simulink model "a_adaptivesInveresFilter"  (R2024b)
settings: Solver=ode45  StartTime=0.0  StopTime=100000.0  RelTol=1e-3  EnableMultiTasking=on
undefined symbols (not defined in the file): Amplitudengang, dspblkCoreblockFVToolHelper, gcbh, Koeffizienten, LMS, RLS
libraries: simulink x3, dspadpt3 x2, dspspect3 x2
settings Model: Creator=Wirnitzer  LastModifiedBy=49179
settings SolverCC: AlgebraicLoopSolver=TrustRegion
settings DataIOCC: LimitDataPoints=on  SaveFormat=Array  SignalLoggingSaveFormat=ModelDataLogs  ReturnWorkspaceOutputs=off
settings OptimizationCC: BooleanDataType=off  InitFltsAndDblsToZero=on  LifeSpan=inf
settings DebuggingCC: SaveWithParameterizedLinksMsg=none  UnderspecifiedInitializationDetection=Classic  MergeDetectMultiDrivingBlocksExec=none  SignalResolutionControl=TryResolveAllWithWarning  MultiTaskDSMMsg=warning  MultiTaskCondExecSysMsg=none  FcnCallInpInsideContextMsg=warning  UnconnectedInputMsg=warning  UnconnectedOutputMsg=warning  UnconnectedLineMsg=warning  SFUnexpectedBacktrackingDiag=warning  SFNoUnconditionalDefaultTransitionDiag=warning  SFExecutionAtInitializationDiag=none  ArithmeticOperatorsInVariantConditions=warning
settings HardwareCC: ProdBitPerPointer=32  ProdBitPerSizeT=32  ProdBitPerPtrDiffT=32  ProdLargestAtomicFloat=None  ProdIntDivRoundTo=Undefined  ProdEndianess=Unspecified  ProdWordSize=32  ProdHWDeviceType=32-bit Generic  TargetUnknown=on
settings ModelReferenceCC: EnableRefExpFcnMdlSchedulingChecks=on  PropagateSignalLabelsOutOfModel=off
settings SFSimCC: CustomCodeUndefinedFunction=UseInterfaceOnly
settings RTWCC: GPUComputeCapability=3.5
settings CodeAppCC: StateflowObjectComments=on
settings GRTTargetCC: TargetFcnLib=ansi_tfl_tmw.mat  TargetLangStandard=C89/C90 (ANSI)  ModelReferenceCompliant=off  CombineOutputUpdateFcns=off  MatFileLogging=off  GRTInterface=on
settings ConfigComp: CovMetricSettings=dw  CovSaveCumulativeToWorkspaceVar=on  CovSaveSingleToWorkspaceVar=on

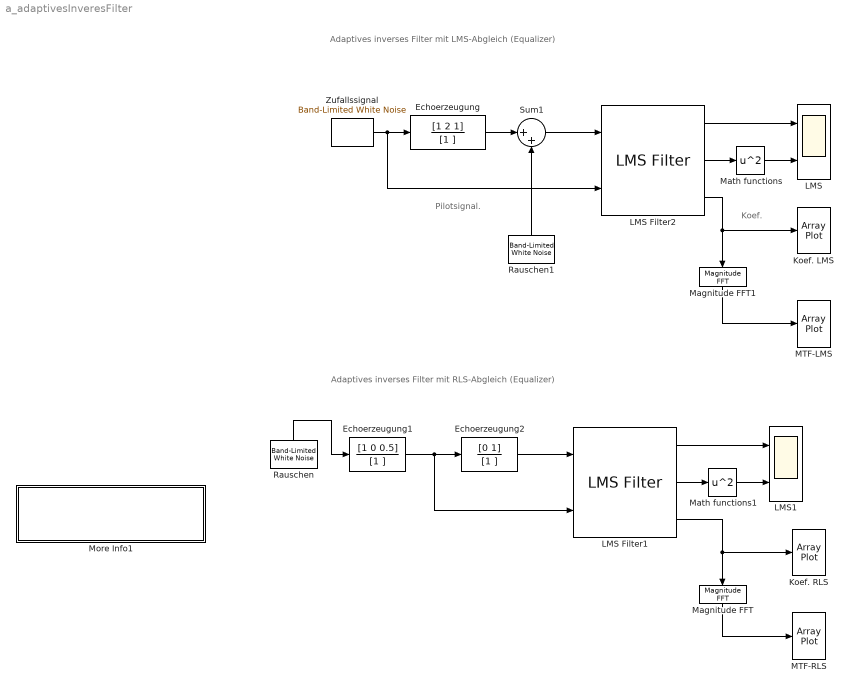
== system a_adaptivesInveresFilter ==
  note: Pilotsignal.
  note: Adaptives inverses  Filter mit RLS-Abgleich
      |  (Equalizer)
  note: Koef.
  note: Adaptives inverses  Filter mit LMS-Abgleich
      | (Equalizer)
  Echoerzeugung : DiscreteFilter  LoadFcn=dspblkCoreblockFVToolHelper(gcbh,'load');  Numerator=[1 2 1]  Denominator=[1 ]  SampleTime=1
      settings: CopyFcn=dspblkCoreblockFVToolHelper(gcbh,'copy');  DeleteFcn=dspblkCoreblockFVToolHelper(gcbh,'close');  ModelCloseFcn=dspblkCoreblockFVToolHelper(gcbh,'close');  PreSaveFcn=dspblkCoreblockFVToolHelper(gcbh,'presave');  PostSaveFcn=dspblkCoreblockFVToolHelper(gcbh,'postsave');  CloseFcn=dspblkCoreblockFVToolHelper(gcbh,'close');
  Echoerzeugung1 : DiscreteFilter  LoadFcn=dspblkCoreblockFVToolHelper(gcbh,'load');  Numerator=[1 0 0.5]  Denominator=[1 ]  SampleTime=1
      settings: CopyFcn=dspblkCoreblockFVToolHelper(gcbh,'copy');  DeleteFcn=dspblkCoreblockFVToolHelper(gcbh,'close');  ModelCloseFcn=dspblkCoreblockFVToolHelper(gcbh,'close');  PreSaveFcn=dspblkCoreblockFVToolHelper(gcbh,'presave');  PostSaveFcn=dspblkCoreblockFVToolHelper(gcbh,'postsave');  CloseFcn=dspblkCoreblockFVToolHelper(gcbh,'close');
  Echoerzeugung2 : DiscreteFilter  LoadFcn=dspblkCoreblockFVToolHelper(gcbh,'load');  Numerator=[0 1]  Denominator=[1 ]  SampleTime=1
      settings: CopyFcn=dspblkCoreblockFVToolHelper(gcbh,'copy');  DeleteFcn=dspblkCoreblockFVToolHelper(gcbh,'close');  ModelCloseFcn=dspblkCoreblockFVToolHelper(gcbh,'close');  PreSaveFcn=dspblkCoreblockFVToolHelper(gcbh,'presave');  PostSaveFcn=dspblkCoreblockFVToolHelper(gcbh,'postsave');  CloseFcn=dspblkCoreblockFVToolHelper(gcbh,'close');
  Koef. LMS : ArrayPlot  WindowPosition=[107.000000,93.000000,450.000000,360.000000,]  Visible=on  ScopeFrameLocation=window  PlotType=Line  AxesScaling=Manual  MaximizeAxes=Off  XLabel=Index  YLabel=LMS-Koeffizienten  YLimits=[-0.48731,0.83885]  ShowGrid=off  ChannelNames="[\"\"]"  DefaultConfigurationName=dsp.scopes.ArrayPlotBlockSpecification
  Koef. RLS : ArrayPlot  WindowPosition=[491.000000,123.000000,450.000000,360.000000,]  Visible=on  ScopeFrameLocation=window  PlotType=Line  AxesScaling=Manual  MaximizeAxes=Off  XLabel=Index  YLabel=RLS-Koeffizienten  YLimits=[-0.42569,0.37868]  ShowGrid=off  ChannelNames="[\"\"]"  DefaultConfigurationName=dsp.scopes.ArrayPlotBlockSpecification
  LMS : Scope  NumInputPorts=2
      settings: AttributesFormatString=test
  LMS Filter1 : dspadpt3/LMS Filter  Algo=Normalized LMS  L=11  stepflag=Dialog  mu=0.005  leakage=1.0  ic=0  Adapt=off  resetflag=None  weights=on  addnparflag=off  roundingMode=Floor  overflowMode=off  secondCoeffMode=Binary point scaling  secondCoeffWordLength=2  secondCoeffFracLength=15  prodOutput2Mode=Binary point scaling  prodOutput2FracLength=20  prodOutput3Mode=Binary point scaling  prodOutput3FracLength=20  prodOutput4Mode=Binary point scaling  prodOutput4FracLength=20  quotientMode=Binary point scaling  quotientFracLength=20  accum2Mode=Binary point scaling  accum2FracLength=20
  LMS Filter2 : dspadpt3/LMS Filter  Algo=Normalized LMS  L=11  stepflag=Dialog  mu=0.05  leakage=1.0  ic=0  Adapt=off  resetflag=None  weights=on  addnparflag=off  roundingMode=Floor  overflowMode=off  secondCoeffMode=Binary point scaling  secondCoeffWordLength=2  secondCoeffFracLength=15  prodOutput2Mode=Binary point scaling  prodOutput2FracLength=20  prodOutput3Mode=Binary point scaling  prodOutput3FracLength=20  prodOutput4Mode=Binary point scaling  prodOutput4FracLength=20  quotientMode=Binary point scaling  quotientFracLength=20  accum2Mode=Binary point scaling  accum2FracLength=20
  LMS1 : Scope  NumInputPorts=2
      settings: AttributesFormatString=test
  MTF-LMS : ArrayPlot  WindowPosition=[401.000000,50.000000,610.000000,635.000000,]  Visible=on  ScopeFrameLocation=window  PlotType=Line  AxesScaling=Manual  MaximizeAxes=Off  XLabel=Frequenzzahl  YLabel=LMS-Amplitudengang  YLimits=[0.46544,1.6287]  ShowGrid=off  ChannelNames="[\"\"]"  DefaultConfigurationName=dsp.scopes.ArrayPlotBlockSpecification
  MTF-RLS : ArrayPlot  WindowPosition=[491.000000,123.000000,764.000000,360.000000,]  Visible=on  ScopeFrameLocation=window  PlotType=Line  AxesScaling=Manual  MaximizeAxes=Off  XLabel=Frequenzzahl  YLabel=RLS-Amplitudengang  YLimits=[0.1012,1.3433]  ShowGrid=off  ChannelNames="[\"\"]"  DefaultConfigurationName=dsp.scopes.ArrayPlotBlockSpecification
  Magnitude FFT : dspspect3/Magnitude FFT  mag_or_magsq=Magnitude  FFTImplementation=Auto  fftLenInherit=off  fftsize=256  WrapInput=on
  Magnitude FFT1 : dspspect3/Magnitude FFT  mag_or_magsq=Magnitude  FFTImplementation=Auto  fftLenInherit=off  fftsize=256  WrapInput=on
  Math functions : Math  Operator=square  SignedPower=on
  Math functions1 : Math  Operator=square  SignedPower=on
  More Info1 : Subsystem
      mask Display: disp(' Aufgaben')
  Rauschen : simulink/Sources/Band-Limited White Noise  Cov=0.3  Ts=1  seed=[241]
  Rauschen1 : simulink/Sources/Band-Limited White Noise  Cov=0.3  Ts=1  seed=[241]
  Sum1 : Sum  Inputs=|++  InputSameDT=on  SaturateOnIntegerOverflow=on  OutDataTypeStr=Inherit: Same as first input
  Zufallssignal : simulink/Sources/Band-Limited White Noise  Cov=1  Ts=1  seed=[23341]
  wires:
  Math functions/1 -> LMS/2
  LMS Filter2/1 -> LMS/1
  LMS Filter2/2 -> Math functions/1
  LMS Filter2/3 -> Koef. LMS/1, Magnitude FFT1/1
  Zufallssignal/1 -> LMS Filter2/2, Echoerzeugung/1
  Math functions1/1 -> LMS1/2
  LMS Filter1/2 -> Math functions1/1
  LMS Filter1/3 -> Koef. RLS/1, Magnitude FFT/1
  Magnitude FFT/1 -> MTF-RLS/1
  Magnitude FFT1/1 -> MTF-LMS/1
  Rauschen/1 -> Echoerzeugung1/1
  Echoerzeugung1/1 -> LMS Filter1/2, Echoerzeugung2/1
  Echoerzeugung2/1 -> LMS Filter1/1
  LMS Filter1/1 -> LMS1/1
  Echoerzeugung/1 -> Sum1/1
  Sum1/1 -> LMS Filter2/1
  Rauschen1/1 -> Sum1/2

== system a_adaptivesInveresFilter/More Info1 ==
  note: Adaptives Inverses System (== Entzerrer == Equalizer)
      | ===========================================
      | (c) HSM, B. Wir 7.11 97, 8.8.2012
      |
      |
      | Starten Sie die Simulation mit  SIMULATION, START.
      | Beobachten Sie wie sich die Koeffizienten des Filters langsam einstellen.
      | Durch einen Doppelklick auf das Oszilloskop können Sie die Signale
      | beobachten. Mit der rechten Maustate können Sie AUTOSCALE aktivieren.
      |
      | (i)   Stellen sich die erwarteten Filterkoeffizienten ein?
      |
      | (ii)  Welche Einflüsse haben die Filterordnung und die Schrittweite des LMS auf das Ergebnis?
      |
      | (iii) Addieren Sie Rauschen zum System und untersuchen Sie (i) und (ii).
      |
      | (iv) Welche Vorteile bringt der RLS-Algorithmus?
      |
      | (v)  Entzerren Sie den Übertragungskanal \( G(z) = 1 + 2z^{-1} + z^{-3} \) und beantworten Sie (i)-(iv).
